simulink model "simulink_4_balloons_nointeraction"  (R2020b)
settings: Solver=VariableStepAuto  StartTime=0.0  StopTime=300  RelTol=1e-3
InitFcn:
  | seed1 = randi(100000);
  | seed2 = randi(200000);
values from neighbouring files (symbols this model uses):
  Cd = 0.185    [sim_1balloon.m]    (also in sim_1balloon_test.m; sim_2balloon.m; sim_2balloon_test.m; sim_4balloon.m)
  mb1 = 3/1000    (= 0.003)    [sim_1balloon.m]    (also in sim_1balloon_test.m; sim_2balloon.m; sim_2balloon_test.m; sim_4balloon.m)
  mb2 = 3/1000    (= 0.003)    [sim_2balloon.m]    (also in sim_2balloon_test.m; sim_4balloon.m; sim_4balloon_test.m)
  mb3 = 3/1000    (= 0.003)    [sim_4balloon.m]    (also in sim_4balloon_test.m)
  mb4 = 3/1000    (= 0.003)    [sim_4balloon.m]    (also in sim_4balloon_test.m)
  nH = optimizableVariable('nH',nHB)    [optimiseB2.m]    (also in optimiseB4.m; sim_1balloon.m = x(2); sim_1balloon_test.m = x(2); sim_2balloon.m = x(2))
  normalScaling = optimizableVariable('normalScaling',normalScalingB)    [optimiseB2.m]    (also in optimiseB4.m; sim_1balloon.m = x(5); sim_1balloon_test.m = x(5); sim_2balloon.m = x(5))
  nS = optimizableVariable('nS',nSB)    [optimiseB2.m]    (also in optimiseB4.m; sim_1balloon.m = x(3); sim_1balloon_test.m = x(3); sim_2balloon.m = x(3))
  nV = optimizableVariable('nV',nVB)    [optimiseB2.m]    (also in optimiseB4.m; sim_1balloon.m = x(1); sim_1balloon_test.m = x(1); sim_2balloon.m = x(1))
  rb1 = 80/1000    (= 0.08)    [sim_1balloon.m]    (also in sim_1balloon_test.m; sim_2balloon.m; sim_2balloon_test.m; sim_4balloon.m)
  rb2 = 80/1000    (= 0.08)    [sim_2balloon.m]    (also in sim_2balloon_test.m; sim_4balloon.m; sim_4balloon_test.m)
  rb3 = 80/1000    (= 0.08)    [sim_4balloon.m]    (also in sim_4balloon_test.m)
  rb4 = 80/1000    (= 0.08)    [sim_4balloon.m]    (also in sim_4balloon_test.m)
  rn = 125/2000    (= 0.0625)    [sim_1balloon.m]    (also in sim_1balloon_test.m; sim_2balloon.m; sim_2balloon_test.m; sim_4balloon.m)
  seedX1 = randi(100000)    [sim_1balloon.m]    (also in sim_1balloon_test.m = x(8); sim_2balloon.m; sim_2balloon_test.m = x(11); sim_4balloon.m)
  seedX2 = randi(100000)    [sim_2balloon.m]    (also in sim_2balloon_test.m = x(14); sim_4balloon.m; sim_4balloon_test.m = x(14))
  seedX3 = randi(100000)    [sim_4balloon.m]    (also in sim_4balloon_test.m = x(17))
  seedX4 = randi(100000)    [sim_4balloon.m]    (also in sim_4balloon_test.m = x(20))
  seedY1 = randi(100000)    [sim_1balloon.m]    (also in sim_1balloon_test.m = x(9); sim_2balloon.m; sim_2balloon_test.m = x(12); sim_4balloon.m)
  seedY2 = randi(100000)    [sim_2balloon.m]    (also in sim_2balloon_test.m = x(15); sim_4balloon.m; sim_4balloon_test.m = x(15))
  seedY3 = randi(100000)    [sim_4balloon.m]    (also in sim_4balloon_test.m = x(18))
  seedY4 = randi(100000)    [sim_4balloon.m]    (also in sim_4balloon_test.m = x(21))
  seedZ1 = randi(100000)    [sim_1balloon.m]    (also in sim_1balloon_test.m = x(10); sim_2balloon.m; sim_2balloon_test.m = x(13); sim_4balloon.m)
  seedZ2 = randi(100000)    [sim_2balloon.m]    (also in sim_2balloon_test.m = x(16); sim_4balloon.m; sim_4balloon_test.m = x(16))
  seedZ3 = randi(100000)    [sim_4balloon.m]    (also in sim_4balloon_test.m = x(19))
  seedZ4 = randi(100000)    [sim_4balloon.m]    (also in sim_4balloon_test.m = x(22))
  theta = optimizableVariable('theta',thetaB)    [optimiseB2.m]    (also in optimiseB4.m; sim_1balloon.m = x(7); sim_1balloon_test.m = x(7); sim_2balloon.m = x(7))
  V0 = optimizableVariable('V0',V0B)    [optimiseB1.m]    (also in optimiseB2.m; optimiseB4.m; sim_1balloon.m = x(4); sim_1balloon_test.m = x(4))
libraries: nesl_utility x41, sm_lib x25, eeGeneralControl x12
(part 2 of 2)

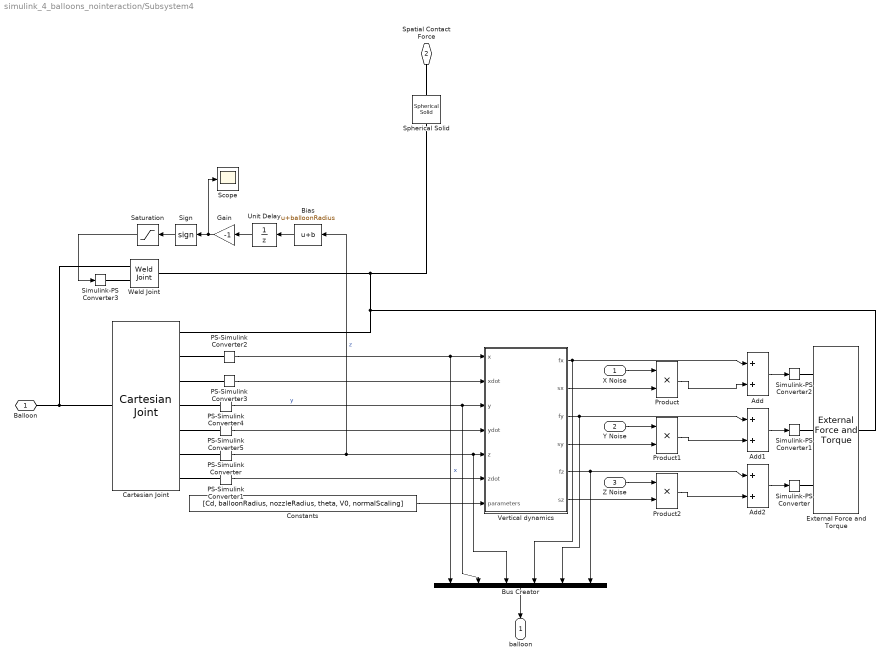
== system simulink_4_balloons_nointeraction/Subsystem4 ==
  X Noise : Inport
  Y Noise : Inport  Port=2
  Z Noise : Inport  Port=3
  Add : Sum
  Add1 : Sum
  Add2 : Sum
  Bias : Bias  Bias=balloonRadius
  Bus Creator : BusCreator  Inputs=6
  Cartesian Joint : sm_lib/Joints/Cartesian Joint  JointMode=Normal  SenseConstraintForce=off  SenseConstraintForceX=off  SenseConstraintForceY=off  SenseConstraintForceZ=off  SenseConstraintTorque=off  SenseConstraintTorqueX=off  SenseConstraintTorqueY=off  SenseConstraintTorqueZ=off  SenseTotalForce=off  SenseTotalForceX=off  SenseTotalForceY=off  SenseTotalForceZ=off  SenseTotalTorque=off  SenseTotalTorqueX=off  SenseTotalTorqueY=off  SenseTotalTorqueZ=off  CompositeWrenchDir=FollowerOnBase  CompositeWrenchFrame=BaseFrame  PxEquilibriumPosition=0  PxEquilibriumPositionUnits=m  PxSpringStiffness=0  PxSpringStiffnessUnits=N/m  PxDampingCoefficient=hd  PxDampingCoefficientUnits=N/(m/s)  PxTorqueActuationMode=NoTorque  PxMotionActuationMode=ComputedMotion  PxSensePosition=on  PxSenseVelocity=on  PxSenseAcceleration=off  PxSenseTorqueForce=off  PxSenseLowerLimitTorqueForce=off  PxSenseUpperLimitTorqueForce=off  PxLowerLimitSpecify=off  PxLowerLimitBound=-1  PxLowerLimitBoundUnits=m  PxLowerLimitStiffness=1e6  PxLowerLimitStiffnessUnits=N/m  PxLowerLimitDamping=1e3  PxLowerLimitDampingUnits=N/(m/s)  PxLowerLimitTransitionRegionWidth=1e-4  PxLowerLimitTransitionRegionWidthUnits=m  PxUpperLimitSpecify=off  PxUpperLimitBound=1  PxUpperLimitBoundUnits=m  PxUpperLimitStiffness=1e6  PxUpperLimitStiffnessUnits=N/m  PxUpperLimitDamping=1e3  PxUpperLimitDampingUnits=N/(m/s)  PxUpperLimitTransitionRegionWidth=1e-4  PxUpperLimitTransitionRegionWidthUnits=m  PxPositionTargetSpecify=off  PxPositionTargetPriority=High  PxPositionTargetValue=0  PxPositionTargetValueUnits=m  PxVelocityTargetSpecify=off  PxVelocityTargetPriority=High  PxVelocityTargetValue=0  PxVelocityTargetValueUnits=m/s  PyEquilibriumPosition=0  PyEquilibriumPositionUnits=m  PySpringStiffness=0  PySpringStiffnessUnits=N/m  PyDampingCoefficient=hd  PyDampingCoefficientUnits=N/(m/s)  PyTorqueActuationMode=NoTorque  PyMotionActuationMode=ComputedMotion  PySensePosition=on  PySenseVelocity=on  PySenseAcceleration=off  PySenseTorqueForce=off  PySenseLowerLimitTorqueForce=off  PySenseUpperLimitTorqueForce=off  PyLowerLimitSpecify=off  PyLowerLimitBound=-1  PyLowerLimitBoundUnits=m  PyLowerLimitStiffness=1e6  PyLowerLimitStiffnessUnits=N/m  PyLowerLimitDamping=1e3  PyLowerLimitDampingUnits=N/(m/s)  PyLowerLimitTransitionRegionWidth=1e-4  PyLowerLimitTransitionRegionWidthUnits=m  PyUpperLimitSpecify=off  PyUpperLimitBound=1  PyUpperLimitBoundUnits=m  PyUpperLimitStiffness=1e6  PyUpperLimitStiffnessUnits=N/m  PyUpperLimitDamping=1e3  PyUpperLimitDampingUnits=N/(m/s)  PyUpperLimitTransitionRegionWidth=1e-4  PyUpperLimitTransitionRegionWidthUnits=m  PyPositionTargetSpecify=off  PyPositionTargetPriority=High  PyPositionTargetValue=0  PyPositionTargetValueUnits=m  PyVelocityTargetSpecify=off  PyVelocityTargetPriority=High  PyVelocityTargetValue=0  PyVelocityTargetValueUnits=m/s  PzEquilibriumPosition=0  PzEquilibriumPositionUnits=m  PzSpringStiffness=0  PzSpringStiffnessUnits=N/m  PzDampingCoefficient=hd  PzDampingCoefficientUnits=N/(m/s)  PzTorqueActuationMode=NoTorque  PzMotionActuationMode=ComputedMotion  PzSensePosition=on  PzSenseVelocity=on  PzSenseAcceleration=off  PzSenseTorqueForce=off  PzSenseLowerLimitTorqueForce=off  PzSenseUpperLimitTorqueForce=off  PzLowerLimitSpecify=off  PzLowerLimitBound=0  PzLowerLimitBoundUnits=m  PzLowerLimitStiffness=1e6  PzLowerLimitStiffnessUnits=N/m  PzLowerLimitDamping=1e3  PzLowerLimitDampingUnits=N/(m/s)  PzLowerLimitTransitionRegionWidth=1e-4  PzLowerLimitTransitionRegionWidthUnits=m  PzUpperLimitSpecify=off  PzUpperLimitBound=1  PzUpperLimitBoundUnits=m  PzUpperLimitStiffness=1e6  PzUpperLimitStiffnessUnits=N/m  PzUpperLimitDamping=1e3  PzUpperLimitDampingUnits=N/(m/s)  PzUpperLimitTransitionRegionWidth=1e-4  PzUpperLimitTransitionRegionWidthUnits=m  PzPositionTargetSpecify=on  PzPositionTargetPriority=High  PzPositionTargetValue=initialHeight  PzPositionTargetValueUnits=m  PzVelocityTargetSpecify=on  PzVelocityTargetPriority=High  PzVelocityTargetValue=0  PzVelocityTargetValueUnits=m/s
  Constants : Constant  Value=[Cd, balloonRadius, nozzleRadius, theta, V0, normalScaling]
  External Force and Torque : sm_lib/Forces and Torques/External Force and Torque  ForceResolutionFrame=AttachedFrame  EnableForceX=on  EnableForceY=on  EnableForceZ=on  EnableForce=off  TorqueResolutionFrame=AttachedFrame  EnableTorqueX=off  EnableTorqueY=off  EnableTorqueZ=off  EnableTorque=off
  Gain : Gain  Gain=-1
  PS-Simulink Converter{,1..5} (6 alike) : nesl_utility/PS-Simulink Converter  PhysicalDomain=network_engine_domain  SubClassName=ps_output  LeftPortType=input  RightPortType=output  PseudoPeriodic=off  Frequencies=[]  Unit=inherit  AffineConversion=off
  Product : Product
  Product1 : Product
  Product2 : Product
  Saturation : Saturate  UpperLimit=0  LowerLimit=-1
  Scope : Scope
  Sign : Signum
  Simulink-PS Converter{,1..3} (4 alike) : nesl_utility/Simulink-PS Converter  PhysicalDomain=network_engine_domain  SubClassName=ps_input  LeftPortType=input  RightPortType=output  PseudoPeriodic=off  Frequencies=[]  NoiseDistribution=none  NoiseParameters=[]  Unit=1  AffineConversion=off  FilteringAndDerivatives=provide  SimscapeFilterOrder=1  InputFilterTimeConstant=0.001  UdotUserProvided=0
  Spherical Solid : sm_lib/Body Elements/Spherical Solid  GraphicAmbientColor=[0.15 0.15 0.15 1.0]  BasedOnType=Mass  CenterOfMass=[0 0 0]  CenterOfMassUnits=m  GraphicDiffuseColor=[1.0 1.0 0.0]  Density=1000  DensityUnits=kg/m^3  DoExposeReferenceFrame=on  GraphicEmissiveColor=[0.0 0.0 0.0 1.0]  ExportEntireGeometry=on  SerializedExposedGeometries=<ExposedGeometries><ExposedGeometry><RawGeometryId>entire</RawGeometryId><ExposedGeometryId>G</ExposedGeometryId></ExposedGeometry></ExposedGeometries>  SerializedFrames=<Frames/>  MarkerShape=Sphere  MarkerSize=10  GraphicType=FromGeometry  InertiaType=CalculateFromGeometry  Mass=balloonMass  MassUnits=kg  MomentsOfInertia=[1 1 1]  MomentsOfInertiaUnits=kg*m^2  GraphicOpacity=1.0  ProductsOfInertia=[0 0 0]  ProductsOfInertiaUnits=kg*m^2  GraphicShininess=75  GraphicSpecularColor=[0.5 0.5 0.5 1.0]  SphereRadius=balloonRadius  SphereRadiusUnits=m  GraphicVisPropType=SimpleVisualProperties
  Unit Delay : UnitDelay  InitialCondition=initialHeight+balloonRadius  SampleTime=0.01  HasFrameUpgradeWarning=on
  Vertical dynamics : MATLAB Function  TreatAsAtomicUnit=on
  Weld Joint : sm_lib/Joints/Weld Joint  JointMode=ProvidedByInput  SenseConstraintForce=off  SenseConstraintForceX=off  SenseConstraintForceY=off  SenseConstraintForceZ=off  SenseConstraintTorque=off  SenseConstraintTorqueX=off  SenseConstraintTorqueY=off  SenseConstraintTorqueZ=off  SenseTotalForce=off  SenseTotalForceX=off  SenseTotalForceY=off  SenseTotalForceZ=off  SenseTotalTorque=off  SenseTotalTorqueX=off  SenseTotalTorqueY=off  SenseTotalTorqueZ=off  CompositeWrenchDir=FollowerOnBase  CompositeWrenchFrame=BaseFrame
  Balloon : PMIOPort  Side=Left
  Spatial Contact Force : PMIOPort  Port=2  Side=Left
  balloon : Outport
  wires:
  PS-Simulink Converter4/1 -> Vertical dynamics/3(y), Bus Creator/2  "y"
  PS-Simulink Converter2/1 -> Bus Creator/1, Vertical dynamics/1(x)  "x"
  Gain/1 -> Scope/1, Sign/1
  Unit Delay/1 -> Gain/1
  Sign/1 -> Saturation/1
  Saturation/1 -> Simulink-PS Converter3/1
  Bias/1 -> Unit Delay/1
  Product2/1 -> Add2/2
  Vertical dynamics/1(fx) -> Add/1, Bus Creator/4
  Vertical dynamics/5(fz) -> Add2/1, Bus Creator/6
  PS-Simulink Converter/1 -> Bus Creator/3, Vertical dynamics/5(z), Bias/1  "z"
  X Noise/1 -> Product/1
  Vertical dynamics/4(sy) -> Product1/2
  Add1/1 -> Simulink-PS Converter1/1
  Add/1 -> Simulink-PS Converter2/1
  Add2/1 -> Simulink-PS Converter/1
  Vertical dynamics/3(fy) -> Add1/1, Bus Creator/5
  Y Noise/1 -> Product1/1
  Vertical dynamics/2(sx) -> Product/2
  Product1/1 -> Add1/2
  Product/1 -> Add/2
  Vertical dynamics/6(sz) -> Product2/2
  Bus Creator/1 -> balloon/1
  Z Noise/1 -> Product2/1
  PS-Simulink Converter5/1 -> Vertical dynamics/4(ydot)
  PS-Simulink Converter1/1 -> Vertical dynamics/6(zdot)
  PS-Simulink Converter3/1 -> Vertical dynamics/2(xdot)
  Constants/1 -> Vertical dynamics/7(parameters)
  connections:
  PS-Simulink Converter/LConn1 -- Cartesian Joint/RConn6
  PS-Simulink Converter2/LConn1 -- Cartesian Joint/RConn2
  Weld Joint/RConn1 -- Spherical Solid/RConn1 -- External Force and Torque/RConn1 -- Cartesian Joint/RConn1
  Cartesian Joint/LConn1 -- Weld Joint/LConn1 -- Balloon/RConn1
  PS-Simulink Converter5/LConn1 -- Cartesian Joint/RConn5
  Cartesian Joint/RConn4 -- PS-Simulink Converter4/LConn1
  PS-Simulink Converter3/LConn1 -- Cartesian Joint/RConn3
  PS-Simulink Converter1/LConn1 -- Cartesian Joint/RConn7
  Simulink-PS Converter3/RConn1 -- Weld Joint/LConn2
  Spatial Contact Force/RConn1 -- Spherical Solid/LConn1
  Simulink-PS Converter1/RConn1 -- External Force and Torque/LConn2
  Simulink-PS Converter/RConn1 -- External Force and Torque/LConn3
  External Force and Torque/LConn1 -- Simulink-PS Converter2/RConn1

== matlab function simulink_4_balloons_nointeraction/Subsystem2/Vertical dynamics ==
  data: fx output; sx output; fy output; sy output; x input; xdot input; y input; ydot input; z input; fz output; zdot input; parameters input; sz output
function [fx,sx,fy,sy,fz,sz] = fcn(x,xdot,y,ydot,z,zdot,parameters)

Cd = parameters(1);
rb = parameters(2);
rn = parameters(3);
theta = deg2rad(parameters(4)); 
V0 = parameters(5); 
normalScaling = parameters(6); 

%% Vertical forces

%flow radius
rFlow = rn+z*tan(theta);

%Peak flow velocity
meanFlowVelocity = V0*rn^2/(rFlow)^2;

%Velocity under ball
vFlowActual = flowSpeed(meanFlowVelocity,normalScaling*rFlow,x,y);

%Relative
relativeVelocity = vFlowActual - zdot;

%Force
fz = sign(relativeVelocity)*0.5*Cd*pi*rb^2*1.22*relativeVelocity^2;



%% Horizontal XY forces
% Bernoulli's Principle
if x == 0 && y == 0
    fx = 0;
    fy = 0;
else
    direction = [x y];
    distance = norm(direction);
    one_direction = direction/distance;
    inner_position = (distance - rb)*one_direction;
    outer_position = (distance + rb)*one_direction;
    vInner = flowSpeed(meanFlowVelocity,normalScaling*rFlow,inner_position(1),inner_position(2));
    vOuter = flowSpeed(meanFlowVelocity,normalScaling*rFlow,outer_position(1),outer_position(2));
    fH = 0.5*1.22*(vOuter^2 - vInner^2)*pi*rb^2*one_direction;
    fx = fH(1);
    fy = fH(2);
end
% Drag
if xdot == 0 && ydot == 0
else
    vxy = [xdot ydot];
    dragH = 0.5*Cd*pi*rb^2*1.22*(xdot^2 + ydot^2)*vxy/norm(vxy);
    fx = fx - dragH(1);
    fy = fy - dragH(2);
end

%% Force scalings
sx = flowSpeed(meanFlowVelocity,normalScaling*rFlow,x,0)/flowSpeed(meanFlowVelocity,rFlow,0,0);
sy = flowSpeed(meanFlowVelocity,normalScaling*rFlow,0,y)/flowSpeed(meanFlowVelocity,rFlow,0,0);
sz = flowSpeed(meanFlowVelocity,normalScaling*rFlow,x,y)/flowSpeed(meanFlowVelocity,rFlow,0,0);

== matlab function simulink_4_balloons_nointeraction/Subsystem1/Vertical dynamics ==
  data: fx output; sx output; fy output; sy output; x input; xdot input; y input; ydot input; z input; fz output; zdot input; parameters input; sz output
function [fx,sx,fy,sy,fz,sz] = fcn(x,xdot,y,ydot,z,zdot,parameters)

Cd = parameters(1);
rb = parameters(2);
rn = parameters(3);
theta = deg2rad(parameters(4)); 
V0 = parameters(5); 
normalScaling = parameters(6); 

%% Vertical forces

%flow radius
rFlow = rn+z*tan(theta);

%Peak flow velocity
meanFlowVelocity = V0*rn^2/(rFlow)^2;

%Velocity under ball
vFlowActual = flowSpeed(meanFlowVelocity,normalScaling*rFlow,x,y);

%Relative
relativeVelocity = vFlowActual - zdot;

%Force
fz = sign(relativeVelocity)*0.5*Cd*pi*rb^2*1.22*relativeVelocity^2;



%% Horizontal XY forces
% Bernoulli's Principle
if x == 0 && y == 0
    fx = 0;
    fy = 0;
else
    direction = [x y];
    distance = norm(direction);
    one_direction = direction/distance;
    inner_position = (distance - rb)*one_direction;
    outer_position = (distance + rb)*one_direction;
    vInner = flowSpeed(meanFlowVelocity,normalScaling*rFlow,inner_position(1),inner_position(2));
    vOuter = flowSpeed(meanFlowVelocity,normalScaling*rFlow,outer_position(1),outer_position(2));
    fH = 0.5*1.22*(vOuter^2 - vInner^2)*pi*rb^2*one_direction;
    fx = fH(1);
    fy = fH(2);
end
% Drag
if xdot == 0 && ydot == 0
else
    vxy = [xdot ydot];
    dragH = 0.5*Cd*pi*rb^2*1.22*(xdot^2 + ydot^2)*vxy/norm(vxy);
    fx = fx - dragH(1);
    fy = fy - dragH(2);
end

%% Force scalings
sx = flowSpeed(meanFlowVelocity,normalScaling*rFlow,x,0)/flowSpeed(meanFlowVelocity,rFlow,0,0);
sy = flowSpeed(meanFlowVelocity,normalScaling*rFlow,0,y)/flowSpeed(meanFlowVelocity,rFlow,0,0);
sz = flowSpeed(meanFlowVelocity,normalScaling*rFlow,x,y)/flowSpeed(meanFlowVelocity,rFlow,0,0);

== matlab function simulink_4_balloons_nointeraction/Subsystem3/Vertical dynamics ==
  data: fx output; sx output; fy output; sy output; x input; xdot input; y input; ydot input; z input; fz output; zdot input; parameters input; sz output
function [fx,sx,fy,sy,fz,sz] = fcn(x,xdot,y,ydot,z,zdot,parameters)

Cd = parameters(1);
rb = parameters(2);
rn = parameters(3);
theta = deg2rad(parameters(4)); 
V0 = parameters(5); 
normalScaling = parameters(6); 

%% Vertical forces

%flow radius
rFlow = rn+z*tan(theta);

%Peak flow velocity
meanFlowVelocity = V0*rn^2/(rFlow)^2;

%Velocity under ball
vFlowActual = flowSpeed(meanFlowVelocity,normalScaling*rFlow,x,y);

%Relative
relativeVelocity = vFlowActual - zdot;

%Force
fz = sign(relativeVelocity)*0.5*Cd*pi*rb^2*1.22*relativeVelocity^2;



%% Horizontal XY forces
% Bernoulli's Principle
if x == 0 && y == 0
    fx = 0;
    fy = 0;
else
    direction = [x y];
    distance = norm(direction);
    one_direction = direction/distance;
    inner_position = (distance - rb)*one_direction;
    outer_position = (distance + rb)*one_direction;
    vInner = flowSpeed(meanFlowVelocity,normalScaling*rFlow,inner_position(1),inner_position(2));
    vOuter = flowSpeed(meanFlowVelocity,normalScaling*rFlow,outer_position(1),outer_position(2));
    fH = 0.5*1.22*(vOuter^2 - vInner^2)*pi*rb^2*one_direction;
    fx = fH(1);
    fy = fH(2);
end
% Drag
if xdot == 0 && ydot == 0
else
    vxy = [xdot ydot];
    dragH = 0.5*Cd*pi*rb^2*1.22*(xdot^2 + ydot^2)*vxy/norm(vxy);
    fx = fx - dragH(1);
    fy = fy - dragH(2);
end

%% Force scalings
sx = flowSpeed(meanFlowVelocity,normalScaling*rFlow,x,0)/flowSpeed(meanFlowVelocity,rFlow,0,0);
sy = flowSpeed(meanFlowVelocity,normalScaling*rFlow,0,y)/flowSpeed(meanFlowVelocity,rFlow,0,0);
sz = flowSpeed(meanFlowVelocity,normalScaling*rFlow,x,y)/flowSpeed(meanFlowVelocity,rFlow,0,0);

== matlab function simulink_4_balloons_nointeraction/Subsystem4/Vertical dynamics ==
  data: fx output; sx output; fy output; sy output; x input; xdot input; y input; ydot input; z input; fz output; zdot input; parameters input; sz output
function [fx,sx,fy,sy,fz,sz] = fcn(x,xdot,y,ydot,z,zdot,parameters)

Cd = parameters(1);
rb = parameters(2);
rn = parameters(3);
theta = deg2rad(parameters(4)); 
V0 = parameters(5); 
normalScaling = parameters(6); 

%% Vertical forces

%flow radius
rFlow = rn+z*tan(theta);

%Peak flow velocity
meanFlowVelocity = V0*rn^2/(rFlow)^2;

%Velocity under ball
vFlowActual = flowSpeed(meanFlowVelocity,normalScaling*rFlow,x,y);

%Relative
relativeVelocity = vFlowActual - zdot;

%Force
fz = sign(relativeVelocity)*0.5*Cd*pi*rb^2*1.22*relativeVelocity^2;



%% Horizontal XY forces
% Bernoulli's Principle
if x == 0 && y == 0
    fx = 0;
    fy = 0;
else
    direction = [x y];
    distance = norm(direction);
    one_direction = direction/distance;
    inner_position = (distance - rb)*one_direction;
    outer_position = (distance + rb)*one_direction;
    vInner = flowSpeed(meanFlowVelocity,normalScaling*rFlow,inner_position(1),inner_position(2));
    vOuter = flowSpeed(meanFlowVelocity,normalScaling*rFlow,outer_position(1),outer_position(2));
    fH = 0.5*1.22*(vOuter^2 - vInner^2)*pi*rb^2*one_direction;
    fx = fH(1);
    fy = fH(2);
end
% Drag
if xdot == 0 && ydot == 0
else
    vxy = [xdot ydot];
    dragH = 0.5*Cd*pi*rb^2*1.22*(xdot^2 + ydot^2)*vxy/norm(vxy);
    fx = fx - dragH(1);
    fy = fy - dragH(2);
end

%% Force scalings
sx = flowSpeed(meanFlowVelocity,normalScaling*rFlow,x,0)/flowSpeed(meanFlowVelocity,rFlow,0,0);
sy = flowSpeed(meanFlowVelocity,normalScaling*rFlow,0,y)/flowSpeed(meanFlowVelocity,rFlow,0,0);
sz = flowSpeed(meanFlowVelocity,normalScaling*rFlow,x,y)/flowSpeed(meanFlowVelocity,rFlow,0,0);
